simulink subsystem "Local_Control"  (R2022b)
settings: Solver=VariableStepAuto  StartTime=0.0  StopTime=10.0  RelTol=1e-3
settings Model: Creator=USER  LastModifiedBy=USER

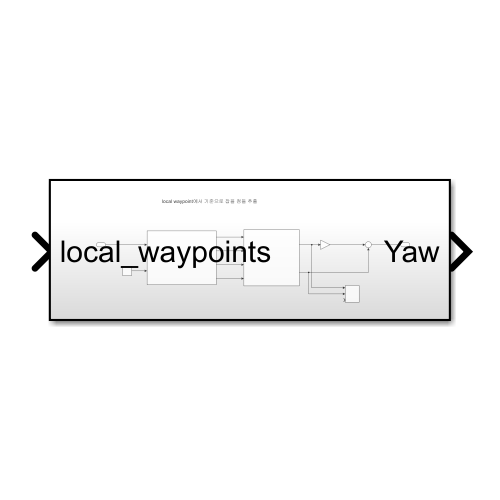
[thumbnail: Simulink's stored preview of the top-level diagram]
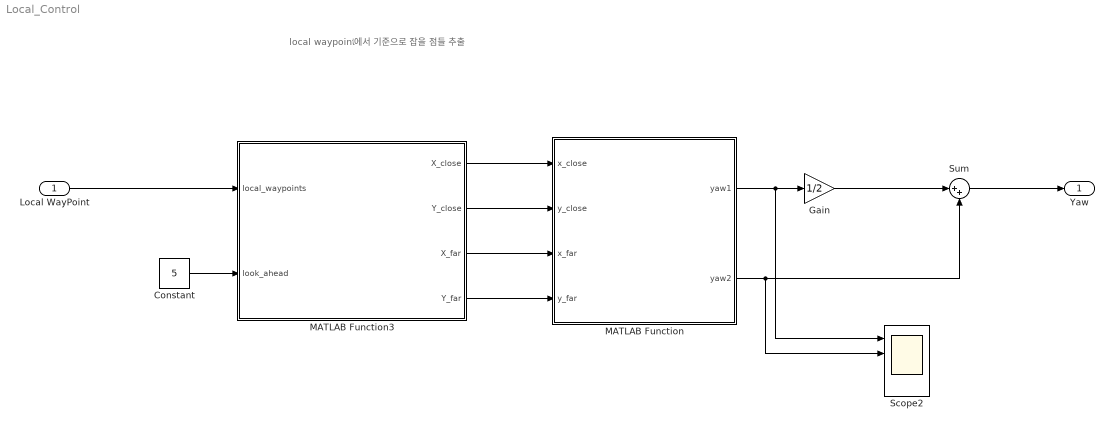
== system Local_Control ==
  note: local waypoint에서 기준으로 잡을 점들 추출
  Local WayPoint : Inport
  Constant : Constant  Value=5
  Gain : Gain  Gain=1/2
  MATLAB Function : MATLAB Function  TreatAsAtomicUnit=on
  MATLAB Function3 : MATLAB Function  TreatAsAtomicUnit=on
  Scope2 : Scope  NumInputPorts=4
  Sum : Sum  Inputs=|++
  Yaw : Outport
  wires:
  Local WayPoint/1 -> MATLAB Function3/1(local_waypoints)
  Sum/1 -> Yaw/1
  MATLAB Function3/1(X_close) -> MATLAB Function/1(x_close)
  MATLAB Function3/2(Y_close) -> MATLAB Function/2(y_close)
  MATLAB Function3/4(Y_far) -> MATLAB Function/4(y_far)
  Gain/1 -> Sum/1
  MATLAB Function/2(yaw2) -> Sum/2, Scope2/2
  Constant/1 -> MATLAB Function3/2(look_ahead)
  MATLAB Function/1(yaw1) -> Scope2/1, Gain/1
  MATLAB Function3/3(X_far) -> MATLAB Function/3(x_far)

== matlab function Local_Control/MATLAB Function ==
  data: x_close input; yaw1 output; y_close input; x_far input; y_far input; yaw2 output
function [yaw1, yaw2] = yaw_calculate(x_close, y_close, x_far, y_far)
    yaw1 = atan2(y_close, 10);
    yaw2 = 0;

    if (x_far ~= 0)&& (y_far ~= 0)
        yaw2 = atan2(y_far, x_far );
    end
end

== matlab function Local_Control/MATLAB Function3 ==
  settings: updateMethod=DISCRETE  sampleTime=0.05
  data: X_close output; Y_close output; local_waypoints input; look_ahead input; X_far output; Y_far output
function [X_close, Y_close, X_far, Y_far] = waypoint_to_xy(local_waypoints, look_ahead)
       
    filtered_matrix = local_waypoints(local_waypoints(:, 1) >= 0, :);
    filtered_matrix = filtered_matrix(filtered_matrix(:, 1) <= 20, :);
    filtered_matrix = filtered_matrix(filtered_matrix(:, 2) >= -20, :);
    filtered_matrix = filtered_matrix(filtered_matrix(:, 2) <= 20, :);
    

    % 3. 5번째 웨이포인트의 X, Y 좌표 가져오기

    X_close = 1;
    Y_close = 0;

    if size(filtered_matrix, 1) > look_ahead
        X_close = filtered_matrix(1, 1);  % 5번째 X 좌표
        Y_close = filtered_matrix(1, 2);  % 5번째 Y 좌표
    end
    
    X_far = 0;
    Y_far = 0;
    
    if size(filtered_matrix, 1) > look_ahead
        X_far = filtered_matrix(look_ahead, 1);
        Y_far = filtered_matrix(look_ahead, 2);
    end
    
end
